simulink model "task2_1"  (R2023b)
settings: Solver=VariableStepAuto  StartTime=0.0  StopTime=10  MaxStep=0.01  RelTol=1e-4  EnableMultiTasking=on
settings Model: Creator=mitcher  LastModifiedBy=mitcher
settings SolverCC: AlgebraicLoopSolver=TrustRegion
settings DataIOCC: LimitDataPoints=on  SaveOutput=off  SaveTime=off
settings OptimizationCC: ExpressionDepthLimit=2147483647  LifeSpan=1
settings DebuggingCC: UnderspecifiedInitializationDetection=Classic  MergeDetectMultiDrivingBlocksExec=none  FcnCallInpInsideContextMsg=warning  UnconnectedInputMsg=warning  UnconnectedOutputMsg=warning  UnconnectedLineMsg=warning  AllowSymbolicDim=off  StateNameClashWarn=warning  SFUnexpectedBacktrackingDiag=warning  SFNoUnconditionalDefaultTransitionDiag=warning  SFExecutionAtInitializationDiag=none  ArithmeticOperatorsInVariantConditions=warning
settings ModelReferenceCC: EnableRefExpFcnMdlSchedulingChecks=on
settings SFSimCC: SimUseLocalCustomCode=off  CustomCodeUndefinedFunction=UseInterfaceOnly
settings RTWCC: RTWUseLocalCustomCode=off
settings CodeAppCC: StateflowObjectComments=on
settings GRTTargetCC: TargetLangStandard=C89/C90 (ANSI)  CombineOutputUpdateFcns=off  GRTInterface=on

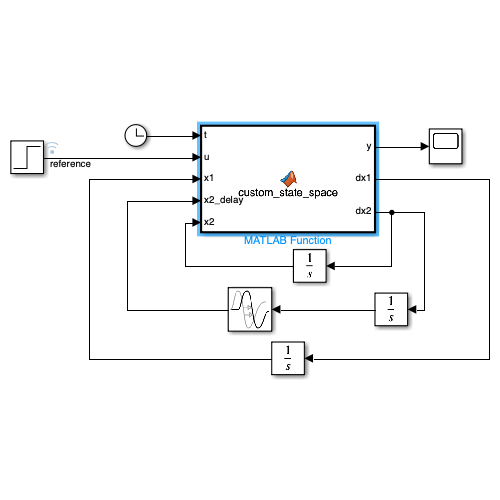
[thumbnail: Simulink's stored preview of the top-level diagram]
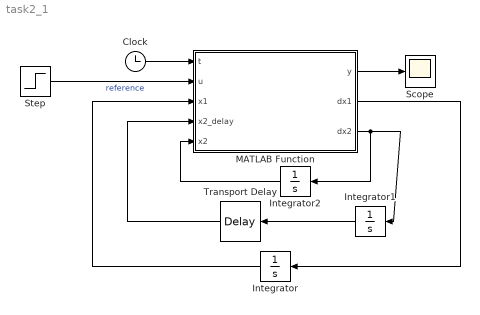
== system task2_1 ==
  Clock : Clock
  Integrator : Integrator
  Integrator1 : Integrator
  Integrator2 : Integrator
  MATLAB Function : MATLAB Function  TreatAsAtomicUnit=on
  Scope : Scope
  Step : Step  Time=1.2  SampleTime=0
  Transport Delay : TransportDelay  DelayTime=0.4
  wires:
  Step/1 -> MATLAB Function/2(u)  "reference"
  MATLAB Function/2(dx1) -> Integrator/1
  Clock/1 -> MATLAB Function/1(t)
  MATLAB Function/1(y) -> Scope/1
  Integrator/1 -> MATLAB Function/3(x1)
  MATLAB Function/3(dx2) -> Integrator2/1, Integrator1/1
  Integrator1/1 -> Transport Delay/1
  Transport Delay/1 -> MATLAB Function/4(x2_delay)
  Integrator2/1 -> MATLAB Function/5(x2)

== matlab function task2_1/MATLAB Function ==
  data: y output; t input; u input; dx1 output; x1 input; x2_delay input; x2 input; dx2 output
function [y, dx1, dx2] = custom_state_space(t, u, x1, x2_delay, x2)
    if t >= 1.4
        dx1 = -4 * x1 + x2_delay;
    else
        dx1 = -4 * x1;
    end

    if t >= 1.2
        dx2 = x1 - 12 * x2 + 3*u;
    else
        dx2 = x1 - 12 * x2;
    end
    y = x1;
